simulink model "Simu_Autopilot_2015_LPF"  (R2024b)
settings: Solver=VariableStepAuto  StartTime=0.0  StopTime=300  FixedStep=0.02  RelTol=1e-3  EnableMultiTasking=on
InitFcn:
  | clear all
  | addpath('../parameters/')
  | aircraft_parameters
  | simulation_parameters
  | wind_parameters
  | compute_autopilot_gains
  | sensor_parameters
undefined symbols (not defined in the file or in its folder): autopilot, drawAircraft, estimate_states_simple, forces_moments, path_follow, path_manager_chap10, plotmavstatevariables, SENSOR, SIM, UAV, WIND
libraries: simulink x6
settings Model: Creator=beard  LastModifiedBy=Administrator
settings SolverCC: AlgebraicLoopSolver=TrustRegion
settings DataIOCC: LimitDataPoints=on  SaveFormat=Array  SignalLoggingSaveFormat=ModelDataLogs  ReturnWorkspaceOutputs=off
settings OptimizationCC: ReuseModelBlockBuffer=off  ExpressionDepthLimit=2147483647  InitFltsAndDblsToZero=on  LifeSpan=inf
settings DebuggingCC: UnderspecifiedInitializationDetection=Classic  MergeDetectMultiDrivingBlocksExec=none  SolverPrmCheckMsg=warning  FcnCallInpInsideContextMsg=warning  UnconnectedInputMsg=warning  UnconnectedOutputMsg=warning  UnconnectedLineMsg=warning  StateNameClashWarn=warning  SFUnexpectedBacktrackingDiag=warning  SFNoUnconditionalDefaultTransitionDiag=warning  SFExecutionAtInitializationDiag=none  ArithmeticOperatorsInVariantConditions=warning
settings HardwareCC: ProdBitPerPointer=32  ProdBitPerSizeT=32  ProdBitPerPtrDiffT=32  ProdLargestAtomicFloat=None  ProdIntDivRoundTo=Undefined  ProdEndianess=Unspecified  ProdWordSize=32  ProdHWDeviceType=32-bit Generic
settings ModelReferenceCC: PropagateSignalLabelsOutOfModel=off
settings SFSimCC: SimUseLocalCustomCode=off  CustomCodeUndefinedFunction=UseInterfaceOnly
settings RTWCC: RTWUseLocalCustomCode=off  GPUComputeCapability=3.5
settings CodeAppCC: StateflowObjectComments=on
settings GRTTargetCC: TargetLangStandard=C89/C90 (ANSI)  CombineOutputUpdateFcns=off  GRTInterface=on
settings ConfigComp: CovMetricSettings=dw  CovSaveCumulativeToWorkspaceVar=on  CovSaveSingleToWorkspaceVar=on  CovExternalEMLEnable=off  CovSFcnEnable=off

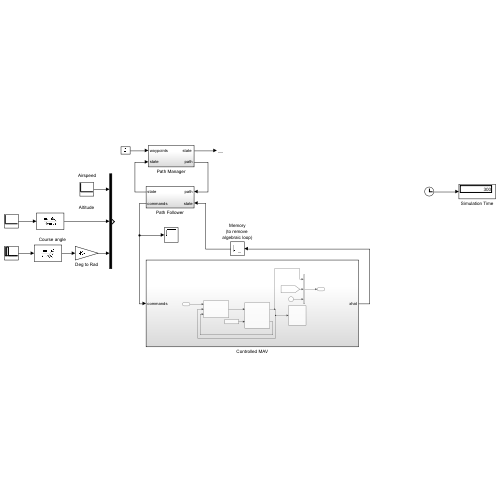
[thumbnail: Simulink's stored preview of the top-level diagram]
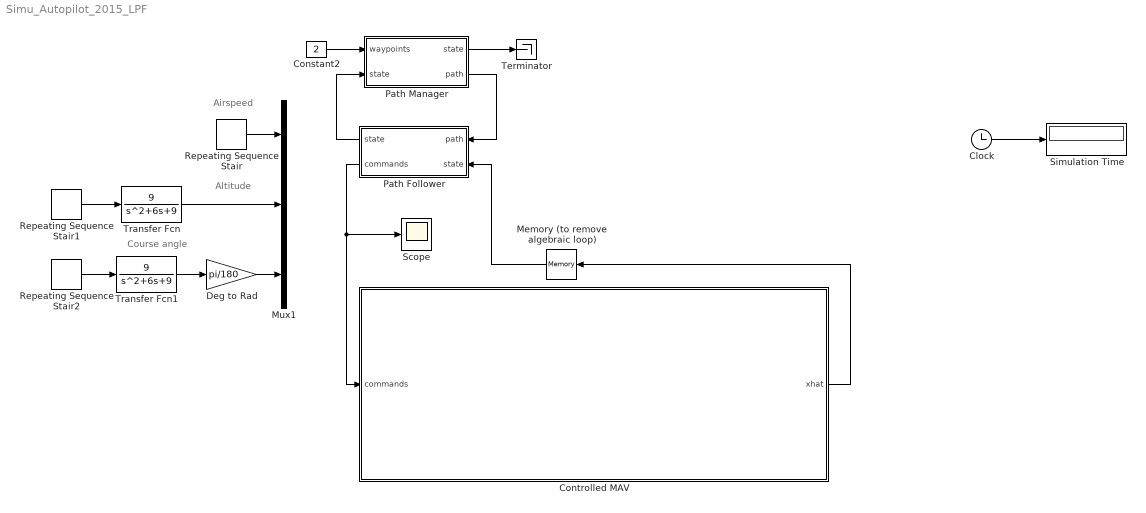
== system Simu_Autopilot_2015_LPF ==
  note: Altitude
  note: Airspeed
  note: Course angle
  Clock : Clock
  Constant2 : Constant  Value=2
  Controlled MAV : Subsystem
  Deg to Rad : Gain  Gain=pi/180
  Memory (to remove algebraic loop) : Memory
  Mux1 : Mux  Inputs=3
  Path Follower : Subsystem
  Path Manager : Subsystem
  Repeating Sequence Stair : simulink/Sources/Repeating Sequence Stair  OutValues=[35].'  tsamp=25  OutMin=[]  OutMax=[]  OutDataTypeStr=double  OutputDataTypeScalingMode=double  OutDataType=fixdt(0,8)  ConRadixGroup=Best Precision: Vector-wise  OutScaling=2^-12
  Repeating Sequence Stair1 : simulink/Sources/Repeating Sequence Stair  OutValues=[10]'  tsamp=25  OutMin=[]  OutMax=[]  OutDataTypeStr=double  OutputDataTypeScalingMode=double  OutDataType=fixdt(0,8)  ConRadixGroup=Best Precision: Vector-wise  OutScaling=2^-12
  Repeating Sequence Stair2 : simulink/Sources/Repeating Sequence Stair  OutValues=[0 10 0 0 0 0 0 0].'  tsamp=25  OutMin=[]  OutMax=[]  OutDataTypeStr=double  OutputDataTypeScalingMode=double  OutDataType=fixdt(0,8)  ConRadixGroup=Best Precision: Vector-wise  OutScaling=2^-12
  Scope : Scope
  Simulation Time : Display
  Terminator : Terminator
  Transfer Fcn : TransferFcn  Numerator=[9]  Denominator=[1 6 9]
  Transfer Fcn1 : TransferFcn  Numerator=[9]  Denominator=[1 6 9]
  wires:
  Clock/1 -> Simulation Time/1
  Deg to Rad/1 -> Mux1/3
  Repeating Sequence Stair1/1 -> Transfer Fcn/1
  Repeating Sequence Stair2/1 -> Transfer Fcn1/1
  Repeating Sequence Stair/1 -> Mux1/1
  Transfer Fcn/1 -> Mux1/2
  Transfer Fcn1/1 -> Deg to Rad/1
  Path Manager/2(path) -> Path Follower/1(path)
  Controlled MAV/1(xhat) -> Memory (to remove algebraic loop)/1
  Path Manager/1("state ") -> Terminator/1
  Path Follower/1("state ") -> Path Manager/2(state)
  Constant2/1 -> Path Manager/1(waypoints)
  Memory (to remove algebraic loop)/1 -> Path Follower/2(state)
  Path Follower/2(commands) -> Controlled MAV/1(commands), Scope/1

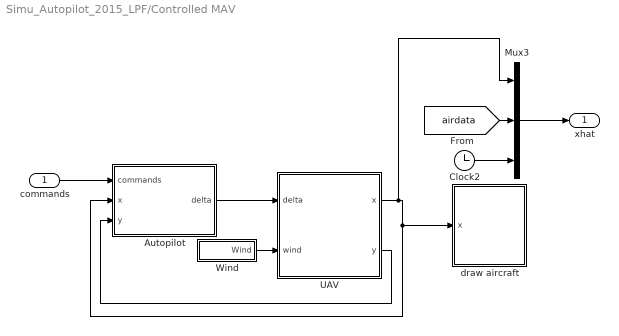
== system Simu_Autopilot_2015_LPF/Controlled MAV ==
  commands : Inport
  Autopilot : Subsystem
      mask Display: image(imread('kestrel.jpg'))
  Clock2 : Clock
  Mux3 : Mux  Inputs=3
  UAV : Subsystem
      mask Display: image(imread('batcam.png'))
  Wind : Subsystem
  draw aircraft : Subsystem
      mask Display: image(imread('tv.jpg'))
  xhat : Outport  VectorParamsAs1DForOutWhenUnconnected=off
  wires:
  Wind/1(Wind) -> UAV/2(wind)
  Autopilot/1(delta) -> UAV/1(delta)
  UAV/2(y) -> Autopilot/3(y)
  commands/1 -> Autopilot/1(commands)
  UAV/1(x) -> Mux3/1, draw aircraft/1(x), Autopilot/2(x)
  Clock2/1 -> Mux3/3
  [airdata] -> Mux3/2
  Mux3/1 -> xhat/1

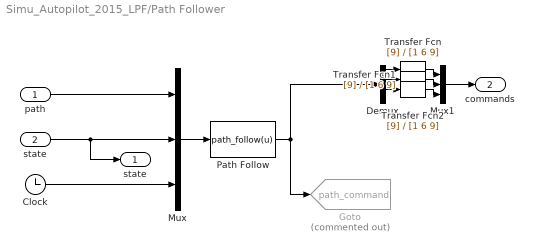
== system Simu_Autopilot_2015_LPF/Path Follower ==
  path : Inport
  state : Inport  Port=2
  Clock : Clock
  Demux : Demux
  Goto : Goto  Commented=on  GotoTag=path_command  TagVisibility=global
  Mux : Mux  Inputs=3
  Mux1 : Mux  Inputs=3
  Path Follow : MATLABFcn  MATLABFcn=path_follow(u)  OutputDimensions=5  SampleTime=SIM.ts_control
  Transfer Fcn : TransferFcn  Numerator=[9]  Denominator=[1 6 9]
  Transfer Fcn1 : TransferFcn  Numerator=[9]  Denominator=[1 6 9]
  Transfer Fcn2 : TransferFcn  Numerator=[9]  Denominator=[1 6 9]
  "state " : Outport  VectorParamsAs1DForOutWhenUnconnected=off
  commands : Outport  Port=2  VectorParamsAs1DForOutWhenUnconnected=off
  wires:
  Path Follow/1 -> Demux/1, Goto/1
  Mux/1 -> Path Follow/1
  path/1 -> Mux/1
  Clock/1 -> Mux/3
  state/1 -> Mux/2, "state "/1
  Demux/1 -> Transfer Fcn/1
  Transfer Fcn/1 -> Mux1/1
  Demux/2 -> Transfer Fcn1/1
  Transfer Fcn1/1 -> Mux1/2
  Transfer Fcn2/1 -> Mux1/3
  Demux/3 -> Transfer Fcn2/1
  Mux1/1 -> commands/1

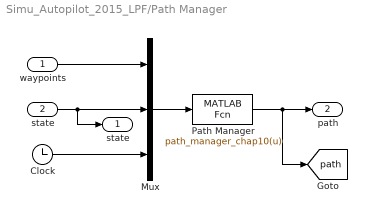
== system Simu_Autopilot_2015_LPF/Path Manager ==
  waypoints : Inport
  state : Inport  Port=2
  Clock : Clock
  Mux : Mux  Inputs=3
  Path Manager : MATLABFcn  MATLABFcn=path_manager_chap10(u)  OutputDimensions=13  SampleTime=SIM.ts_control
  "state " : Outport  VectorParamsAs1DForOutWhenUnconnected=off
  path : Outport  Port=2  VectorParamsAs1DForOutWhenUnconnected=off
  tag scope: path=global
  wires:
  Path Manager/1 -> path/1, [path]
  Mux/1 -> Path Manager/1
  Clock/1 -> Mux/3
  state/1 -> Mux/2, "state "/1
  waypoints/1 -> Mux/1

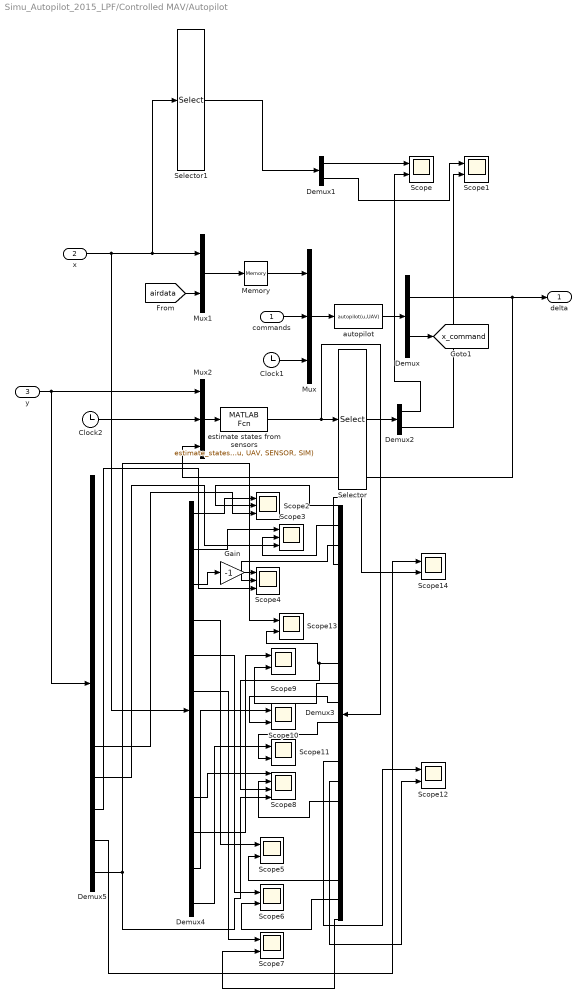
== system Simu_Autopilot_2015_LPF/Controlled MAV/Autopilot ==
  commands : Inport
  x : Inport  Port=2
  y : Inport  Port=3
  Clock1 : Clock
  Clock2 : Clock
  Demux : Demux  Outputs=[4;12]
  Demux1 : Demux  Outputs=2
  Demux2 : Demux  Outputs=2
  Demux3 : Demux  Outputs=22
  Demux4 : Demux  Outputs=12
  Demux5 : Demux  Outputs=13
  Gain : Gain  Gain=-1
  Memory : Memory
  Mux : Mux  Inputs=3
  Mux1 : Mux  Inputs=2
  Mux2 : Mux  Inputs=3
  Scope{,1,5..7,9..14} (11 alike) : Scope  NumInputPorts=2
  Scope2 : Scope  NumInputPorts=3
  Scope3 : Scope  NumInputPorts=3
  Scope4 : Scope  NumInputPorts=3
  Scope8 : Scope  NumInputPorts=4
  Selector : Selector  InputPortWidth=22  IndexOptions=Index vector (dialog)  Indices=[7 8]  OutputSizes=1
  Selector1 : Selector  InputPortWidth=12  IndexOptions=Index vector (dialog)  Indices=[7 8]  OutputSizes=1
  autopilot : MATLABFcn  MATLABFcn=autopilot(u,UAV)  OutputDimensions=4+12  SampleTime=SIM.ts_simulation
  estimate states from sensors : MATLABFcn  MATLABFcn=estimate_states_simple(u, UAV, SENSOR, SIM)  OutputDimensions=22  SampleTime=SIM.ts_control
  delta : Outport
  tag scope: x_command=global
  wires:
  Mux/1 -> autopilot/1
  autopilot/1 -> Demux/1
  Demux/1 -> Mux2/3, delta/1
  Demux/2 -> [x_command]
  commands/1 -> Mux/2
  y/1 -> Demux5/1, Mux2/1
  [airdata] -> Mux1/2
  Clock1/1 -> Mux/3
  Mux1/1 -> Memory/1
  Memory/1 -> Mux/1
  Clock2/1 -> Mux2/2
  Mux2/1 -> estimate states from sensors/1
  x/1 -> Demux4/1, Selector1/1, Mux1/1
  estimate states from sensors/1 -> Demux3/1, Selector/1
  Selector1/1 -> Demux1/1
  Selector/1 -> Demux2/1
  Demux1/1 -> Scope/1
  Demux2/1 -> Scope/2
  Demux1/2 -> Scope1/1
  Demux2/2 -> Scope1/2
  Demux4/1 -> Scope2/1
  Demux3/1 -> Scope2/2
  Demux4/2 -> Scope3/1
  Demux3/2 -> Scope3/2
  Demux3/3 -> Scope4/2
  Gain/1 -> Scope4/1
  Demux4/3 -> Gain/1
  Demux5/9 -> Scope2/3
  Demux5/10 -> Scope3/3
  Demux5/11 -> Scope4/3
  Demux3/20 -> Scope5/2
  Demux4/4 -> Scope5/1
  Demux3/21 -> Scope6/2
  Demux4/5 -> Scope6/1
  Demux3/22 -> Scope7/2
  Demux4/6 -> Scope7/1
  Demux3/16 -> Scope8/2
  Demux4/9 -> Scope8/1
  Demux3/10 -> Scope9/2
  Demux4/10 -> Scope9/1
  Demux3/11 -> Scope10/2
  Demux4/11 -> Scope10/1
  Demux3/12 -> Scope11/2
  Demux4/12 -> Scope11/1
  Demux3/14 -> Scope12/1
  Demux3/15 -> Scope12/2
  Demux3/9 -> Scope8/3, Scope13/2
  Demux5/13 -> Scope13/1, Scope8/4
  Demux3/4 -> Scope14/2
  Demux5/12 -> Scope14/1

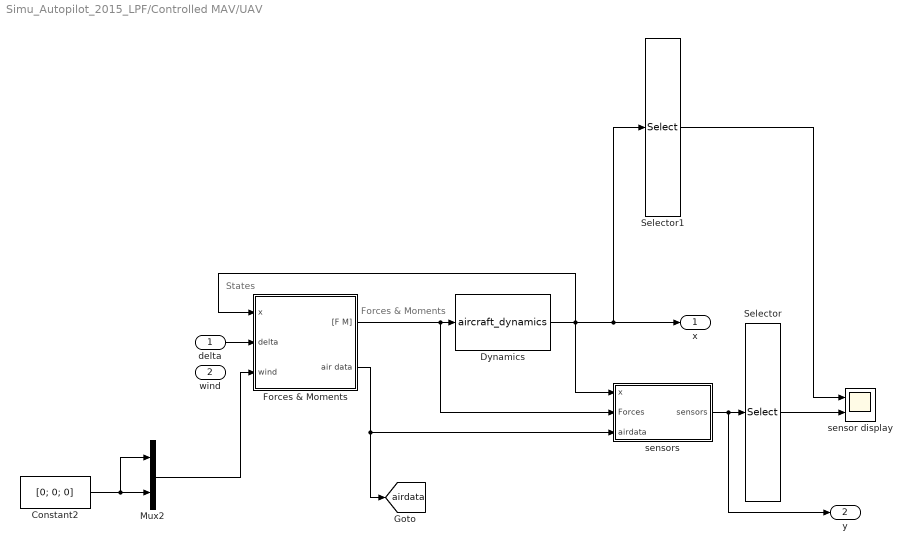
== system Simu_Autopilot_2015_LPF/Controlled MAV/UAV ==
  note: Forces & Moments
  note: States
  delta : Inport
  wind : Inport  Port=2
  Constant2 : Constant  Value=[0; 0; 0]
  Dynamics : S-Function  FunctionName=aircraft_dynamics  Parameters=UAV  SFunctionDeploymentMode=off  EnableBusSupport=off
  Forces & Moments : Subsystem
  Mux2 : Mux  Inputs=2
  Selector : Selector  InputPortWidth=13  IndexOptions=Index vector (dialog)  Indices=[10]  OutputSizes=1
  Selector1 : Selector  InputPortWidth=12  IndexOptions=Index vector (dialog)  Indices=2  OutputSizes=1
  sensor display : Scope  NumInputPorts=2
  sensors : Subsystem
  x : Outport
  y : Outport  Port=2
  tag scope: airdata=global
  wires:
  Forces & Moments/1("[F M]") -> sensors/2(Forces), Dynamics/1
  Forces & Moments/2(air data) -> sensors/3(airdata), [airdata]
  sensors/1(sensors) -> y/1, Selector/1
  Selector/1 -> sensor display/2
  Constant2/1 -> Mux2/1, Mux2/2
  Mux2/1 -> Forces & Moments/3(wind)
  delta/1 -> Forces & Moments/2(delta)
  Dynamics/1 -> sensors/1(x), Selector1/1, x/1, Forces & Moments/1(x)
  Selector1/1 -> sensor display/1

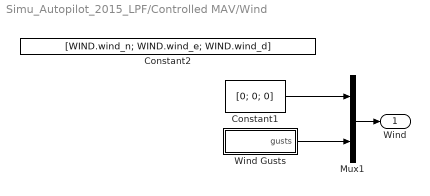
== system Simu_Autopilot_2015_LPF/Controlled MAV/Wind ==
  Constant1 : Constant  Value=[0; 0; 0]
  Constant2 : Constant  Value=[WIND.wind_n; WIND.wind_e; WIND.wind_d]
  Mux1 : Mux  Inputs=2
  Wind Gusts : Subsystem
  Wind : Outport
  wires:
  Mux1/1 -> Wind/1
  Wind Gusts/1(gusts) -> Mux1/2
  Constant1/1 -> Mux1/1

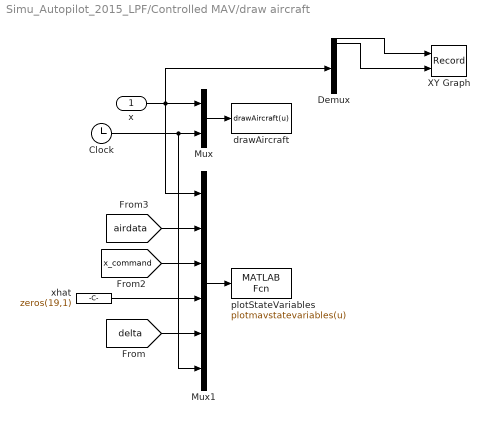
== system Simu_Autopilot_2015_LPF/Controlled MAV/draw aircraft ==
  x : Inport
  Clock : Clock
  Demux : Demux  Outputs=12
  Mux : Mux  Inputs=2
  Mux1 : Mux  Inputs=6
  XY Graph : Record  FileSettingsInternal="{\"entries\":[{\"content\":{\"excelSettings\":{\"content\":{},\"type\":\"Streamout.ExcelSettings\"}},\"type\":\"Streamout.FileSettingStorage\",\"uuid\":\"\"}],\"packageUris\":[\"http:\\/\\/schema.mathworks.com\\/mf0\\/streamout_blocks\\/R2020a\"],\"version\":\"1.0\"}"  Layout=[1 1]  SignalsInternal="{\"entries\":[{\"content\":{\"signals\":[{\"content\":{\"blockPath\":[],\"dimensions\":[1],\"domain\":\"\",\"lineColor\":\"#a2142f\",\"plots\":[ 1 ],\"port\":1,\"sid\":[\"\"],\"signalID\":1,\"signalName\":\"Demux:1\"},\"type\":\"RecordBlkView.Signal\",\"uuid\":\"\"},{\"content\":{\"blockPath\":[],\"dimensions\":[1],\"domain\":\"\",\"lineColor\":\"#139fff\",\"plots\":[ 1 ],\"port\":2,\"sid\":[\"\"],\"signalID\":2,\"signalName\":\"Demux:2\"},\"type\":\"RecordBlkView.Signal\",\"uuid\":\"\"}]},\"type\":\"RecordBlkView.InputSignals\",\"uuid\":\"\"}],\"packageUris\":[\"http:\\/\\/schema.mathworks.com\\/mf0\\/streamout_blocks\\/R2020a\"],\"version\":\"1.0\"}"  VisualizationBindings="{\"xyplotplugin\":{\"info\":[{\"series\":[{\"bindingParametersList\":[{\"parameter\":\"X-Axis\",\"signalID\":1,\"signalName\":\"Demux:1\"},{\"parameter\":\"Y-Axis\",\"signalID\":2,\"signalName\":\"Demux:2\"}],\"seriesID\":0}],\"subplotID\":1}]}}"  CompatibilityTag=XY
  drawAircraft : MATLABFcn  MATLABFcn=drawAircraft(u)  OutputDimensions=0  SampleTime=SIM.ts_plotting
  plotStateVariables : MATLABFcn  MATLABFcn=plotmavstatevariables(u)  OutputDimensions=0  SampleTime=SIM.ts_plotting
  xhat : Constant  Value=zeros(19,1)
  wires:
  Mux/1 -> drawAircraft/1
  Clock/1 -> Mux1/6, Mux/2
  Mux1/1 -> plotStateVariables/1
  [x_command] -> Mux1/3
  [delta] -> Mux1/5
  [airdata] -> Mux1/2
  xhat/1 -> Mux1/4
  Demux/1 -> XY Graph/1
  Demux/2 -> XY Graph/2
  x/1 -> Demux/1, Mux1/1, Mux/1

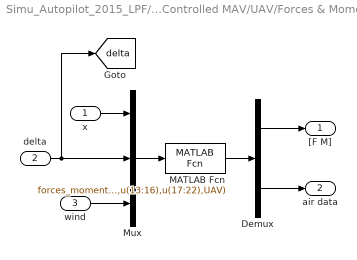
== system Simu_Autopilot_2015_LPF/Controlled MAV/UAV/Forces & Moments ==
  x : Inport
  delta : Inport  Port=2
  wind : Inport  Port=3
  Demux : Demux  Outputs=[6;6]
  MATLAB Fcn : MATLABFcn  MATLABFcn=forces_moments(u(1:12),u(13:16),u(17:22),UAV)  OutputDimensions=12
  Mux : Mux  Inputs=3
  "[F M]" : Outport
  air data : Outport  Port=2
  tag scope: delta=global
  wires:
  Mux/1 -> MATLAB Fcn/1
  Demux/1 -> "[F M]"/1
  MATLAB Fcn/1 -> Demux/1
  wind/1 -> Mux/3
  delta/1 -> [delta], Mux/2
  x/1 -> Mux/1
  Demux/2 -> air data/1

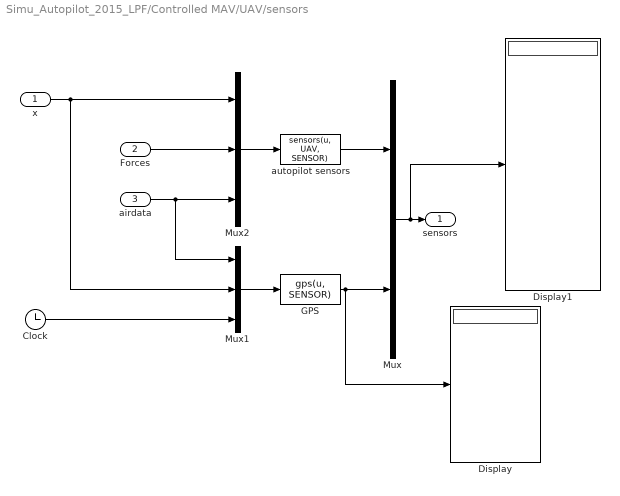
== system Simu_Autopilot_2015_LPF/Controlled MAV/UAV/sensors ==
  x : Inport
  Forces : Inport  Port=2
  airdata : Inport  Port=3
  Clock : Clock
  Display : Display
  Display1 : Display
  GPS : MATLABFcn  MATLABFcn=gps(u, SENSOR)  OutputDimensions=5  SampleTime=SENSOR.ts_gps
  Mux : Mux  Inputs=2
  Mux1 : Mux  Inputs=3
  Mux2 : Mux  Inputs=3
  autopilot sensors : MATLABFcn  MATLABFcn=sensors(u, UAV, SENSOR)  OutputDimensions=8  SampleTime=SIM.ts_simulation
  sensors : Outport
  wires:
  autopilot sensors/1 -> Mux/1
  Mux1/1 -> GPS/1
  Clock/1 -> Mux1/3
  Mux2/1 -> autopilot sensors/1
  Forces/1 -> Mux2/2
  airdata/1 -> Mux2/3, Mux1/1
  Mux/1 -> Display1/1, sensors/1
  GPS/1 -> Display/1, Mux/2
  x/1 -> Mux1/2, Mux2/1

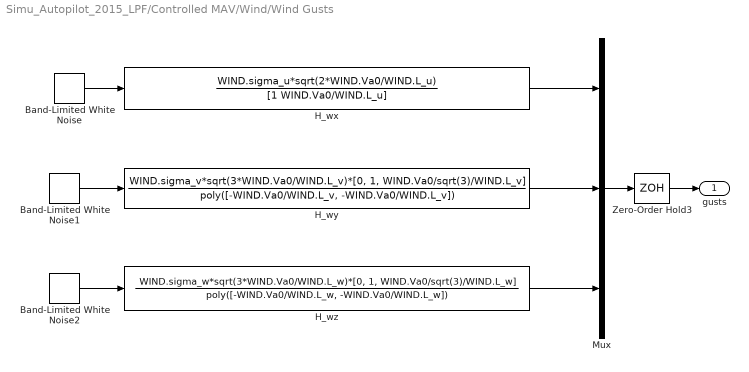
== system Simu_Autopilot_2015_LPF/Controlled MAV/Wind/Wind Gusts ==
  Band-Limited White Noise : simulink/Sources/Band-Limited White Noise  Cov=[0.1]  Ts=SIM.ts_simulation  seed=[23341]
  Band-Limited White Noise1 : simulink/Sources/Band-Limited White Noise  Cov=[0.1]  Ts=SIM.ts_simulation  seed=[23341]
  Band-Limited White Noise2 : simulink/Sources/Band-Limited White Noise  Cov=[0.1]  Ts=SIM.ts_simulation  seed=[23341]
  H_wx : TransferFcn  Numerator=WIND.sigma_u*sqrt(2*WIND.Va0/WIND.L_u)  Denominator=[1 WIND.Va0/WIND.L_u]
  H_wy : TransferFcn  Numerator=WIND.sigma_v*sqrt(3*WIND.Va0/WIND.L_v)*[0, 1, WIND.Va0/sqrt(3)/WIND.L_v]  Denominator=poly([-WIND.Va0/WIND.L_v, -WIND.Va0/WIND.L_v])
  H_wz : TransferFcn  Numerator=WIND.sigma_w*sqrt(3*WIND.Va0/WIND.L_w)*[0, 1, WIND.Va0/sqrt(3)/WIND.L_w]  Denominator=poly([-WIND.Va0/WIND.L_w, -WIND.Va0/WIND.L_w])
  Mux : Mux  Inputs=3
  Zero-Order Hold3 : ZeroOrderHold  SampleTime=SIM.ts_simulation
  gusts : Outport
  wires:
  H_wx/1 -> Mux/1
  Band-Limited White Noise/1 -> H_wx/1
  H_wy/1 -> Mux/2
  Band-Limited White Noise1/1 -> H_wy/1
  H_wz/1 -> Mux/3
  Band-Limited White Noise2/1 -> H_wz/1
  Mux/1 -> Zero-Order Hold3/1
  Zero-Order Hold3/1 -> gusts/1
